simulink model "MIL_ASW"  (R2019b)
settings: Solver=FixedStepDiscrete  StartTime=0.0  StopTime=2  FixedStep=0.001  RelTol=1e-3  EnableMultiTasking=on
model workspace (MAT data in the model file):
  AccPedlCanVal : Simulink.Signal (value not decoded)
  AccPedlVal : Simulink.Signal (value not decoded)
  BrkPedlCanVal : Simulink.Signal (value not decoded)
  BrkPedlVal : Simulink.Signal (value not decoded)
  Cal1 : Simulink.Parameter (value not decoded)
  Cal10 : Simulink.Parameter (value not decoded)
  Cal11 : Simulink.Parameter (value not decoded)
  Cal12 : Simulink.Parameter (value not decoded)
  Cal2 : Simulink.Parameter (value not decoded)
  Cal3 : Simulink.Parameter (value not decoded)
  Cal4 : Simulink.Parameter (value not decoded)
  Cal5 : Simulink.Parameter (value not decoded)
  Cal6 : Simulink.Parameter (value not decoded)
  Cal7 : Simulink.Parameter (value not decoded)
  Cal8 : Simulink.Parameter (value not decoded)
  Cal9 : Simulink.Parameter (value not decoded)
  Clu1Act : Simulink.Signal (value not decoded)
  Clu1PTar : Simulink.Signal (value not decoded)
  Clu1Req : Simulink.Signal (value not decoded)
  Clu1TqTar : Simulink.Signal (value not decoded)
  Clu2Act : Simulink.Signal (value not decoded)
  Clu2PTar : Simulink.Signal (value not decoded)
  Clu2Req : Simulink.Signal (value not decoded)
  Clu2TqTar : Simulink.Signal (value not decoded)
  CluKissPtPLnch : Simulink.Parameter (value not decoded)
  CluOilTRawVal : Simulink.Signal (value not decoded)
  CluOilTVal : Simulink.Signal (value not decoded)
  CluOpenTqRatMax : Simulink.Parameter (value not decoded)
  CluPMap : Simulink.Parameter (value not decoded)
  CluPMax : Simulink.Parameter (value not decoded)
  CluPMaxGear1 : Simulink.Parameter (value not decoded)
  CluPMaxGear2 : Simulink.Parameter (value not decoded)
  CluPMaxGear3 : Simulink.Parameter (value not decoded)
  CluPMaxGear4 : Simulink.Parameter (value not decoded)
  CluPMaxGear5 : Simulink.Parameter (value not decoded)
  CluPMaxGear6 : Simulink.Parameter (value not decoded)
  CluPMaxGearR : Simulink.Parameter (value not decoded)
  CluPMin : Simulink.Parameter (value not decoded)
  CluPosnMax : Simulink.Parameter (value not decoded)
  CluSoln1IRawVal : Simulink.Signal (value not decoded)
  CluSoln1IReq : Simulink.Signal (value not decoded)
  CluSoln1IReqFlg : Simulink.Signal (value not decoded)
  CluSoln1IVal : Simulink.Signal (value not decoded)
  CluSoln1LineI : Simulink.Parameter (value not decoded)
  CluSoln1LineP : Simulink.Parameter (value not decoded)
  CluSoln1Pwm : Simulink.Signal (value not decoded)
  CluSoln2IRawVal : Simulink.Signal (value not decoded)
  CluSoln2IReq : Simulink.Signal (value not decoded)
  CluSoln2IReqFlg : Simulink.Signal (value not decoded)
  CluSoln2IVal : Simulink.Signal (value not decoded)
  CluSoln2LineI : Simulink.Parameter (value not decoded)
  CluSoln2LineP : Simulink.Parameter (value not decoded)
  CluSoln2Pwm : Simulink.Signal (value not decoded)
  CluTqMap : Simulink.Parameter (value not decoded)
  CrnkSpdRawVal : Simulink.Signal (value not decoded)
  CrnkSpdVal : Simulink.Signal (value not decoded)
  Drive_Intensity_Fuzzy : object (value not decoded)
  DrvIntenFzzy : Simulink.LookupTable (value not decoded)
  EngNIdle : Simulink.Parameter (value not decoded)
  EngNIdleMin : Simulink.Parameter (value not decoded)
  EngSpdCanVal : Simulink.Signal (value not decoded)
  EngThrCanVal : Simulink.Signal (value not decoded)
  EngTqAdd : Simulink.Parameter (value not decoded)
  EngTqCanVal : Simulink.Signal (value not decoded)
  EngTqIntvFlg : Simulink.Signal (value not decoded)
  EngTqIntvRat : Simulink.Signal (value not decoded)
  EngTqMapExtChartc : Simulink.Parameter (value not decoded)
  EngTqMapSpdIndx : Simulink.Parameter (value not decoded)
  EngTqMapThrtIndx : Simulink.Parameter (value not decoded)
  EngTqMapTqMax : Simulink.Parameter (value not decoded)
  EngTqMaxNorm : Simulink.Parameter (value not decoded)
  EngTqRef : Simulink.Parameter (value not decoded)
  EvenCluPRawVal : Simulink.Signal (value not decoded)
  EvenCluPVal : Simulink.Signal (value not decoded)
  EvenInpSpdRawVal : Simulink.Signal (value not decoded)
  EvenInpSpdVal : Simulink.Signal (value not decoded)
  FcnCallTime : Simulink.Parameter (value not decoded)
  FinalRat : Simulink.Parameter (value not decoded)
  Fork1A : Simulink.Parameter (value not decoded)
  Fork1Act : Simulink.Signal (value not decoded)
  Fork1B : Simulink.Parameter (value not decoded)
  Fork1DeltaSpdTar : Simulink.Parameter (value not decoded)
  Fork1MaxSpd1A : Simulink.Parameter (value not decoded)
  Fork1MaxSpd1B : Simulink.Parameter (value not decoded)
  Fork1MaxSpd2A : Simulink.Parameter (value not decoded)
  Fork1MaxSpd2B : Simulink.Parameter (value not decoded)
  Fork1PosnA : Simulink.Parameter (value not decoded)
  Fork1PosnB : Simulink.Parameter (value not decoded)
  Fork1PosnMaxSpd1A : Simulink.Parameter (value not decoded)
  Fork1PosnMaxSpd1B : Simulink.Parameter (value not decoded)
  Fork1PosnMaxSpd2A : Simulink.Parameter (value not decoded)
  Fork1PosnMaxSpd2B : Simulink.Parameter (value not decoded)
  Fork1PosnNeut : Simulink.Parameter (value not decoded)
  Fork1PosnNeutA : Simulink.Parameter (value not decoded)
  Fork1PosnNeutB : Simulink.Parameter (value not decoded)
  Fork1PosnRawVal : Simulink.Signal (value not decoded)
  Fork1PosnSyncA : Simulink.Parameter (value not decoded)
  Fork1PosnSyncB : Simulink.Parameter (value not decoded)
  Fork1PosnVal : Simulink.Signal (value not decoded)
  Fork1SyncTar : Simulink.Parameter (value not decoded)
  Fork2A : Simulink.Parameter (value not decoded)
  Fork2Act : Simulink.Signal (value not decoded)
  Fork2B : Simulink.Parameter (value not decoded)
  Fork2DeltaSpdTar : Simulink.Parameter (value not decoded)
  Fork2MaxSpd1A : Simulink.Parameter (value not decoded)
  Fork2MaxSpd1B : Simulink.Parameter (value not decoded)
  Fork2MaxSpd2A : Simulink.Parameter (value not decoded)
  Fork2MaxSpd2B : Simulink.Parameter (value not decoded)
  Fork2PosnA : Simulink.Parameter (value not decoded)
  Fork2PosnB : Simulink.Parameter (value not decoded)
  Fork2PosnMaxSpd1A : Simulink.Parameter (value not decoded)
  Fork2PosnMaxSpd1B : Simulink.Parameter (value not decoded)
  Fork2PosnMaxSpd2A : Simulink.Parameter (value not decoded)
  Fork2PosnMaxSpd2B : Simulink.Parameter (value not decoded)
  Fork2PosnNeut : Simulink.Parameter (value not decoded)
  Fork2PosnNeutA : Simulink.Parameter (value not decoded)
  Fork2PosnNeutB : Simulink.Parameter (value not decoded)
  Fork2PosnRawVal : Simulink.Signal (value not decoded)
  Fork2PosnSyncA : Simulink.Parameter (value not decoded)
  Fork2PosnSyncB : Simulink.Parameter (value not decoded)
  Fork2PosnVal : Simulink.Signal (value not decoded)
  Fork2SyncTar : Simulink.Parameter (value not decoded)
  Fork3A : Simulink.Parameter (value not decoded)
  Fork3Act : Simulink.Signal (value not decoded)
  Fork3B : Simulink.Parameter (value not decoded)
  Fork3DeltaSpdTar : Simulink.Parameter (value not decoded)
  Fork3MaxSpd1A : Simulink.Parameter (value not decoded)
  Fork3MaxSpd1B : Simulink.Parameter (value not decoded)
  Fork3MaxSpd2A : Simulink.Parameter (value not decoded)
  Fork3MaxSpd2B : Simulink.Parameter (value not decoded)
  Fork3PosnA : Simulink.Parameter (value not decoded)
  Fork3PosnB : Simulink.Parameter (value not decoded)
  Fork3PosnMaxSpd1A : Simulink.Parameter (value not decoded)
  Fork3PosnMaxSpd1B : Simulink.Parameter (value not decoded)
  Fork3PosnMaxSpd2A : Simulink.Parameter (value not decoded)
  Fork3PosnMaxSpd2B : Simulink.Parameter (value not decoded)
  Fork3PosnNeut : Simulink.Parameter (value not decoded)
  Fork3PosnNeutA : Simulink.Parameter (value not decoded)
  Fork3PosnNeutB : Simulink.Parameter (value not decoded)
  Fork3PosnRawVal : Simulink.Signal (value not decoded)
  Fork3PosnSyncA : Simulink.Parameter (value not decoded)
  Fork3PosnSyncB : Simulink.Parameter (value not decoded)
  Fork3PosnVal : Simulink.Signal (value not decoded)
  Fork3SyncTar : Simulink.Parameter (value not decoded)
  Fork4A : Simulink.Parameter (value not decoded)
  Fork4Act : Simulink.Signal (value not decoded)
  Fork4B : Simulink.Parameter (value not decoded)
  Fork4DeltaSpdTar : Simulink.Parameter (value not decoded)
  Fork4MaxSpd1A : Simulink.Parameter (value not decoded)
  Fork4MaxSpd1B : Simulink.Parameter (value not decoded)
  Fork4MaxSpd2A : Simulink.Parameter (value not decoded)
  Fork4MaxSpd2B : Simulink.Parameter (value not decoded)
  Fork4PosnA : Simulink.Parameter (value not decoded)
  Fork4PosnB : Simulink.Parameter (value not decoded)
  Fork4PosnMaxSpd1A : Simulink.Parameter (value not decoded)
  Fork4PosnMaxSpd1B : Simulink.Parameter (value not decoded)
  Fork4PosnMaxSpd2A : Simulink.Parameter (value not decoded)
  Fork4PosnMaxSpd2B : Simulink.Parameter (value not decoded)
  Fork4PosnNeut : Simulink.Parameter (value not decoded)
  Fork4PosnNeutA : Simulink.Parameter (value not decoded)
  Fork4PosnNeutB : Simulink.Parameter (value not decoded)
  Fork4PosnRawVal : Simulink.Signal (value not decoded)
  Fork4PosnSyncA : Simulink.Parameter (value not decoded)
  Fork4PosnSyncB : Simulink.Parameter (value not decoded)
  Fork4PosnVal : Simulink.Signal (value not decoded)
  Fork4SyncTar : Simulink.Parameter (value not decoded)
  FrntWhlRd : Simulink.Parameter (value not decoded)
  GearIdx : Simulink.Parameter (value not decoded)
  GearMax : Simulink.Parameter (value not decoded)
  GearRat : Simulink.Parameter (value not decoded)
  Launch_Engage_Fuzzy : object (value not decoded)
  LnchEngmtFzzy : Simulink.LookupTable (value not decoded)
  LubeSolnIRawVal : Simulink.Signal (value not decoded)
  LubeSolnIReq : Simulink.Signal (value not decoded)
  LubeSolnIVal : Simulink.Signal (value not decoded)
  LubeSolnLineI : Simulink.Parameter (value not decoded)
  LubeSolnLineP : Simulink.Parameter (value not decoded)
  LubeSolnPwm : Simulink.Signal (value not decoded)
  MaiLineSolnIRawVal : Simulink.Signal (value not decoded)
  MaiLineSolnIReq : Simulink.Signal (value not decoded)
  MaiLineSolnIVal : Simulink.Signal (value not decoded)
  MaiLineSolnLineI : Simulink.Parameter (value not decoded)
  MaiLineSolnLineP : Simulink.Parameter (value not decoded)
  MaiLineSolnPwm : Simulink.Signal (value not decoded)
  OddCluPRawVal : Simulink.Signal (value not decoded)
  OddCluPVal : Simulink.Signal (value not decoded)
  OddInpSpdRawVal : Simulink.Signal (value not decoded)
  OddInpSpdVal : Simulink.Signal (value not decoded)
  OutpSpdRawVal : Simulink.Signal (value not decoded)
  OutpSpdVal : Simulink.Signal (value not decoded)
  PsnsrLineP : Simulink.Parameter (value not decoded)
  PsnsrLineV : Simulink.Parameter (value not decoded)
  SftLvrCanVal : Simulink.Signal (value not decoded)
  SftLvrCfm : Simulink.Signal (value not decoded)
  SftLvrVal : Simulink.Signal (value not decoded)
  Shaft1GearAct : Simulink.Signal (value not decoded)
  Shaft1GearReq : Simulink.Signal (value not decoded)
  Shaft2GearAct : Simulink.Signal (value not decoded)
  Shaft2GearReq : Simulink.Signal (value not decoded)
  ShiftMux1SwtReq : Simulink.Signal (value not decoded)
  ShiftMux2SwtReq : Simulink.Signal (value not decoded)
  ShiftSdlEcoDwnSeln : Simulink.Parameter (value not decoded)
  ShiftSdlEcoDwnShift : Simulink.Parameter (value not decoded)
  ShiftSdlEcoUpSeln : Simulink.Parameter (value not decoded)
  ShiftSdlEcoUpShift : Simulink.Parameter (value not decoded)
  ShiftSdlPwrDwnSeln : Simulink.Parameter (value not decoded)
  ShiftSdlPwrDwnShift : Simulink.Parameter (value not decoded)
  ShiftSdlPwrUpSeln : Simulink.Parameter (value not decoded)
  ShiftSdlPwrUpShift : Simulink.Parameter (value not decoded)
  ShiftSdlSACDwnSeln : Simulink.Parameter (value not decoded)
  ShiftSdlSACDwnShift : Simulink.Parameter (value not decoded)
  ShiftSdlSACUpSeln : Simulink.Parameter (value not decoded)
  ShiftSdlSACUpShift : Simulink.Parameter (value not decoded)
  ShiftSdlThrPedlIdx : Simulink.Parameter (value not decoded)
  ShiftSoln1IRawVal : Simulink.Signal (value not decoded)
  ShiftSoln1IReq : Simulink.Signal (value not decoded)
  ShiftSoln1IVal : Simulink.Signal (value not decoded)
  ShiftSoln1LineI : Simulink.Parameter (value not decoded)
  ShiftSoln1LineP : Simulink.Parameter (value not decoded)
  ShiftSoln1Pwm : Simulink.Signal (value not decoded)
  ShiftSoln2IRawVal : Simulink.Signal (value not decoded)
  ShiftSoln2IReq : Simulink.Signal (value not decoded)
  ShiftSoln2IVal : Simulink.Signal (value not decoded)
  ShiftSoln2LineI : Simulink.Parameter (value not decoded)
  ShiftSoln2LineP : Simulink.Parameter (value not decoded)
  ShiftSoln2Pwm : Simulink.Signal (value not decoded)
  SolnOutpTRawVal : Simulink.Signal (value not decoded)
  SolnOutpTVal : Simulink.Signal (value not decoded)
  TSnsr1LineR : Simulink.Parameter (value not decoded)
  TSnsr2LineR : Simulink.Parameter (value not decoded)
  TrsmNrGearAct : Simulink.Signal (value not decoded)
  TrsmNrGearReq : Simulink.Signal (value not decoded)
  TrsmNrPreGearAct : Simulink.Signal (value not decoded)
  TrsmNrPreGearReq : Simulink.Signal (value not decoded)
  Tsnsr1LineT : Simulink.Parameter (value not decoded)
  Tsnsr2LineT : Simulink.Parameter (value not decoded)
  VehSpdCanVal : Simulink.Signal (value not decoded)
  VehSpdTrsmEstimd : Simulink.Signal (value not decoded)
  VehSpdVal : Simulink.Signal (value not decoded)
  VlvBodyTRawVal : Simulink.Signal (value not decoded)
  VlvBodyTVal : Simulink.Signal (value not decoded)
symbols that are objects in the model workspace (value not decoded): CluPMap, CluSoln1LineI, CluSoln1LineP, CluSoln2LineI, CluSoln2LineP, CluTqMap, EngNIdle, EngNIdleMin, EngTqMapThrtIndx, EngTqMapTqMax, EngTqMaxNorm, FcnCallTime, FinalRat, Fork1A, Fork1B, Fork1DeltaSpdTar, Fork1PosnA, Fork1PosnB, Fork1PosnMaxSpd1A, Fork1PosnMaxSpd1B, Fork1PosnMaxSpd2A, Fork1PosnMaxSpd2B, Fork1PosnNeut, Fork1PosnNeutA, Fork1PosnNeutB, Fork1PosnSyncA, Fork1PosnSyncB, Fork1SyncTar, Fork2A, Fork2B, Fork2DeltaSpdTar, Fork2PosnA, Fork2PosnB, Fork2PosnMaxSpd1A, Fork2PosnMaxSpd1B, Fork2PosnMaxSpd2A, Fork2PosnMaxSpd2B, Fork2PosnNeut, Fork2PosnNeutA, Fork2PosnNeutB, Fork2PosnSyncA, Fork2PosnSyncB, Fork2SyncTar, Fork3A, Fork3B, Fork3DeltaSpdTar, Fork3PosnA, Fork3PosnB, Fork3PosnMaxSpd1A, Fork3PosnMaxSpd1B, Fork3PosnMaxSpd2A, Fork3PosnMaxSpd2B, Fork3PosnNeut, Fork3PosnNeutA, Fork3PosnNeutB, Fork3PosnSyncA, Fork3PosnSyncB, Fork3SyncTar, Fork4A, Fork4B
undefined symbols (not defined in the file or in its folder): in1, out1
libraries: simulink x44, fuzblock x3
(part 6 of 10)

== system MIL_ASW/Application_Software_SHAW/ASW_DrivingStrategy/Auto_Mode_Decision/SptMod ==
  AccPedlVal : Inport
  TrsmPreNrGearAct : Inport  Port=2
  TrsmNrGearAct : Inport  Port=3
  Constant : Constant  Value=30000  OutDataTypeStr=uint16
  Constant1 : Constant  Value=0  OutDataTypeStr=uint16
  Constant2 : Constant  Value=30000  OutDataTypeStr=uint16
  Constant3 : Constant  Value=0  OutDataTypeStr=uint16
  Interval Test : simulink/Logic and Bit Operations/Interval Test  IntervalClosedRight=on  uplimit=GearMax-1  IntervalClosedLeft=on  lowlimit=1  OutDataTypeStr=uint8
  Interval Test1 : simulink/Logic and Bit Operations/Interval Test  IntervalClosedRight=on  uplimit=GearMax  IntervalClosedLeft=on  lowlimit=2  OutDataTypeStr=uint8
  Interval Test2 : simulink/Logic and Bit Operations/Interval Test  IntervalClosedRight=on  uplimit=GearMax-1  IntervalClosedLeft=on  lowlimit=1  OutDataTypeStr=uint8
  Interval Test3 : simulink/Logic and Bit Operations/Interval Test  IntervalClosedRight=on  uplimit=GearMax  IntervalClosedLeft=on  lowlimit=2  OutDataTypeStr=uint8
  Saturation : Saturate  UpperLimit=GearMax-1  LowerLimit=1  OutDataTypeStr=uint8
  Saturation1 : Saturate  UpperLimit=GearMax  LowerLimit=2  OutDataTypeStr=uint8
  Saturation2 : Saturate  UpperLimit=GearMax-1  LowerLimit=1  OutDataTypeStr=uint8
  Saturation3 : Saturate  UpperLimit=GearMax  LowerLimit=2  OutDataTypeStr=uint8
  Select{1..4} (4 alike) : Switch  Criteria=u2 ~= 0
  ShiftSdlPwrDwnSeln : Lookup_n-D  BreakpointsForDimension1=ShiftSdlThrPedlIdx  BreakpointsForDimension2=GearIdx  Table=ShiftSdlPwrDwnSeln  TableDataTypeStr=uint16  ExtrapMethod=Clip  OutDataTypeStr=Inherit: Inherit from 'Table data'  RndMeth=Simplest  InputSameDT=on
  ShiftSdlPwrDwnShift : Lookup_n-D  BreakpointsForDimension1=ShiftSdlThrPedlIdx  BreakpointsForDimension2=GearIdx  Table=ShiftSdlPwrDwnShift  TableDataTypeStr=uint16  ExtrapMethod=Clip  OutDataTypeStr=Inherit: Inherit from 'Table data'  RndMeth=Simplest  InputSameDT=on
  ShiftSdlPwrUpSeln : Lookup_n-D  BreakpointsForDimension1=ShiftSdlThrPedlIdx  BreakpointsForDimension2=GearIdx  Table=ShiftSdlPwrUpSeln  TableDataTypeStr=uint16  ExtrapMethod=Clip  OutDataTypeStr=Inherit: Inherit from 'Table data'  RndMeth=Simplest  InputSameDT=on
  ShiftSdlPwrUpShift : Lookup_n-D  BreakpointsForDimension1=ShiftSdlThrPedlIdx  BreakpointsForDimension2=GearIdx  Table=ShiftSdlPwrUpShift  TableDataTypeStr=uint16  ExtrapMethod=Clip  OutDataTypeStr=Inherit: Inherit from 'Table data'  RndMeth=Simplest  InputSameDT=on
  u-1 : Subsystem
  u-2 : Subsystem
  UpSeln : Outport  VectorParamsAs1DForOutWhenUnconnected=off
  DwnSeln : Outport  Port=2  VectorParamsAs1DForOutWhenUnconnected=off
  UpShift : Outport  Port=3  VectorParamsAs1DForOutWhenUnconnected=off
  DwnShift : Outport  Port=4  VectorParamsAs1DForOutWhenUnconnected=off
  wires:
  TrsmPreNrGearAct/1 -> Saturation/1, Interval Test/1, Saturation1/1, Interval Test1/1
  u-1/1(Out) -> ShiftSdlPwrDwnShift/2
  u-2/1(Out) -> ShiftSdlPwrDwnSeln/2
  AccPedlVal/1 -> ShiftSdlPwrDwnSeln/1, ShiftSdlPwrUpShift/1, ShiftSdlPwrDwnShift/1, ShiftSdlPwrUpSeln/1
  ShiftSdlPwrUpSeln/1 -> Select1/1
  ShiftSdlPwrDwnSeln/1 -> Select2/1
  ShiftSdlPwrUpShift/1 -> Select3/1
  ShiftSdlPwrDwnShift/1 -> Select4/1
  Interval Test/1 -> Select1/2
  Interval Test1/1 -> Select2/2
  Interval Test2/1 -> Select3/2
  Interval Test3/1 -> Select4/2
  Constant/1 -> Select1/3
  Constant1/1 -> Select2/3
  Constant2/1 -> Select3/3
  Constant3/1 -> Select4/3
  Select1/1 -> UpSeln/1
  Select2/1 -> DwnSeln/1
  Select3/1 -> UpShift/1
  Select4/1 -> DwnShift/1
  Saturation/1 -> ShiftSdlPwrUpSeln/2
  Saturation2/1 -> ShiftSdlPwrUpShift/2
  Saturation1/1 -> u-2/1(In)
  Saturation3/1 -> u-1/1(In)
  TrsmNrGearAct/1 -> Interval Test2/1, Saturation3/1, Interval Test3/1, Saturation2/1

== system MIL_ASW/Application_Software_SHAW/ASW_DrivingStrategy/Auto_Mode_Decision/TrsmNrGearTarCalcnAutMod/Upshift_Frozen ==
  acc_pedl : Inport  OutDataTypeStr=uint8
  brk_pedl : Inport  Port=2  OutDataTypeStr=uint8
  veh_spd : Inport  Port=3  OutDataTypeStr=uint16
  f : TriggerPort  TriggerType=function-call  VariantControl=(inherit)
      settings: CopyFcn=Stateflow.SLINSF.SimulinkMan.removeBlockPreDeleteFcn  PreDeleteFcn=Stateflow.SLINSF.SimulinkMan.unsafePredeleteFcn
  Compare To Zero : simulink/Logic and Bit Operations/Compare To Zero  relop=<=  OutDataTypeStr=boolean
  Compare To Zero1 : simulink/Logic and Bit Operations/Compare To Zero  relop=>  OutDataTypeStr=boolean
  Constant : Constant  OutDataTypeStr=uint8
  Constant1 : Constant  Value=0  OutDataTypeStr=uint8
  Delay : Delay  DelayLength=1  InitialCondition=0
  Delay1 : Delay  InitialCondition=0
  Delay2 : Delay  DelayLength=10  InitialCondition=0
  Logical Operator : Logic  Operator=OR  Inputs=3  AllPortsSameDT=off  OutDataTypeStr=boolean
  Logical Operator1 : Logic  Operator=OR  Inputs=3  AllPortsSameDT=off  OutDataTypeStr=boolean
  Logical Operator2 : Logic  Operator=NOR  Inputs=3  AllPortsSameDT=off  OutDataTypeStr=boolean
  Relational Operator : RelationalOperator  Operator=<  OutDataTypeStr=boolean  RndMeth=Simplest
  Relational Operator1 : RelationalOperator  Operator=<  OutDataTypeStr=boolean  RndMeth=Simplest
  Relational Operator2 : RelationalOperator  Operator=<  OutDataTypeStr=boolean  RndMeth=Simplest
  Switch : Switch  Criteria=u2 > Threshold
  Switch1 : Switch  Criteria=u2 > Threshold
  Terminator : Terminator
  Unit Delay1 : UnitDelay  SampleTime=-1  HasFrameUpgradeWarning=on
  flag : Outport  OutDataTypeStr=uint8  VectorParamsAs1DForOutWhenUnconnected=off
  wires:
  Delay/1 -> Relational Operator/2
  Switch/1 -> Unit Delay1/1, flag/1
  Constant/1 -> Switch/1
  Switch1/1 -> Switch/3
  veh_spd/1 -> Terminator/1
  Logical Operator2/1 -> Switch1/2
  Constant1/1 -> Switch1/1
  Unit Delay1/1 -> Switch1/3
  Delay1/1 -> Relational Operator1/2
  Delay2/1 -> Relational Operator2/2
  acc_pedl/1 -> Relational Operator2/1, Compare To Zero/1, Delay2/1, Delay1/1, Relational Operator1/1, Delay/1, Relational Operator/1
  Relational Operator/1 -> Logical Operator/1
  Relational Operator1/1 -> Logical Operator/2
  Relational Operator2/1 -> Logical Operator/3
  Compare To Zero/1 -> Logical Operator2/2, Logical Operator1/2
  brk_pedl/1 -> Compare To Zero1/1
  Logical Operator/1 -> Logical Operator2/1, Logical Operator1/1
  Compare To Zero1/1 -> Logical Operator2/3, Logical Operator1/3
  Logical Operator1/1 -> Switch/2

== system MIL_ASW/Application_Software_SHAW/ASW_GearPositioner/Fork1/Ini_ForkAct/position_A ==
  In1 : Inport
  Action Port : ActionPort  ActionPortLabel=elseif(u1>u2)
  Out1 : Outport  VectorParamsAs1DForOutWhenUnconnected=off
  wires:
  In1/1 -> Out1/1

== system MIL_ASW/Application_Software_SHAW/ASW_GearPositioner/Fork1/Ini_ForkAct/position_B ==
  In1 : Inport
  Action Port : ActionPort  ActionPortLabel=elseif( u1<u5)
  Out1 : Outport  VectorParamsAs1DForOutWhenUnconnected=off
  wires:
  In1/1 -> Out1/1

== system MIL_ASW/Application_Software_SHAW/ASW_GearPositioner/Fork1/Ini_ForkAct/position_between_Neutral_A ==
  In1 : Inport
  Action Port : ActionPort  ActionPortLabel=elseif( u1<=u2&u1>u3)
  Out1 : Outport  VectorParamsAs1DForOutWhenUnconnected=off
  wires:
  In1/1 -> Out1/1

== system MIL_ASW/Application_Software_SHAW/ASW_GearPositioner/Fork1/Ini_ForkAct/position_between_Neutral_B ==
  In1 : Inport
  Action Port : ActionPort  ActionPortLabel=elseif( u1<u4&u1>=u5)
  Out1 : Outport  VectorParamsAs1DForOutWhenUnconnected=off
  wires:
  In1/1 -> Out1/1

== system MIL_ASW/Application_Software_SHAW/ASW_GearPositioner/Fork1/Ini_ForkAct/position_neutral ==
  In1 : Inport
  Action Port : ActionPort  ActionPortLabel=if(u1<=u3&u1>=u4)
  Out1 : Outport  VectorParamsAs1DForOutWhenUnconnected=off
  wires:
  In1/1 -> Out1/1

== system MIL_ASW/Application_Software_SHAW/ASW_GearPositioner/Fork2/Ini_ForkAct/position_A ==
  In1 : Inport
  Action Port : ActionPort  ActionPortLabel=elseif(u1>u2)
  Out1 : Outport  VectorParamsAs1DForOutWhenUnconnected=off
  wires:
  In1/1 -> Out1/1

== system MIL_ASW/Application_Software_SHAW/ASW_GearPositioner/Fork2/Ini_ForkAct/position_B ==
  In1 : Inport
  Action Port : ActionPort  ActionPortLabel=elseif( u1<u5)
  Out1 : Outport  VectorParamsAs1DForOutWhenUnconnected=off
  wires:
  In1/1 -> Out1/1

== system MIL_ASW/Application_Software_SHAW/ASW_GearPositioner/Fork2/Ini_ForkAct/position_between_Neutral_A ==
  In1 : Inport
  Action Port : ActionPort  ActionPortLabel=elseif( u1<=u2&u1>u3)
  Out1 : Outport  VectorParamsAs1DForOutWhenUnconnected=off
  wires:
  In1/1 -> Out1/1

== system MIL_ASW/Application_Software_SHAW/ASW_GearPositioner/Fork2/Ini_ForkAct/position_between_Neutral_B ==
  In1 : Inport
  Action Port : ActionPort  ActionPortLabel=elseif( u1<u4&u1>=u5)
  Out1 : Outport  VectorParamsAs1DForOutWhenUnconnected=off
  wires:
  In1/1 -> Out1/1

== system MIL_ASW/Application_Software_SHAW/ASW_GearPositioner/Fork2/Ini_ForkAct/position_neutral ==
  In1 : Inport
  Action Port : ActionPort  ActionPortLabel=if(u1<=u3&u1>=u4)
  Out1 : Outport  VectorParamsAs1DForOutWhenUnconnected=off
  wires:
  In1/1 -> Out1/1

== system MIL_ASW/Application_Software_SHAW/ASW_GearPositioner/Fork3/Ini_ForkAct/position_A ==
  In1 : Inport
  Action Port : ActionPort  ActionPortLabel=elseif(u1>u2)
  Out1 : Outport  VectorParamsAs1DForOutWhenUnconnected=off
  wires:
  In1/1 -> Out1/1

== system MIL_ASW/Application_Software_SHAW/ASW_GearPositioner/Fork3/Ini_ForkAct/position_B ==
  In1 : Inport
  Action Port : ActionPort  ActionPortLabel=elseif( u1<u5)
  Out1 : Outport  VectorParamsAs1DForOutWhenUnconnected=off
  wires:
  In1/1 -> Out1/1

== system MIL_ASW/Application_Software_SHAW/ASW_GearPositioner/Fork3/Ini_ForkAct/position_between_Neutral_A ==
  In1 : Inport
  Action Port : ActionPort  ActionPortLabel=elseif( u1<=u2&u1>u3)
  Out1 : Outport  VectorParamsAs1DForOutWhenUnconnected=off
  wires:
  In1/1 -> Out1/1

== system MIL_ASW/Application_Software_SHAW/ASW_GearPositioner/Fork3/Ini_ForkAct/position_between_Neutral_B ==
  In1 : Inport
  Action Port : ActionPort  ActionPortLabel=elseif( u1<u4&u1>=u5)
  Out1 : Outport  VectorParamsAs1DForOutWhenUnconnected=off
  wires:
  In1/1 -> Out1/1

== system MIL_ASW/Application_Software_SHAW/ASW_GearPositioner/Fork3/Ini_ForkAct/position_neutral ==
  In1 : Inport
  Action Port : ActionPort  ActionPortLabel=if(u1<=u3&u1>=u4)
  Out1 : Outport  VectorParamsAs1DForOutWhenUnconnected=off
  wires:
  In1/1 -> Out1/1

== system MIL_ASW/Application_Software_SHAW/ASW_GearPositioner/Fork4/Ini_ForkAct/position_A ==
  In1 : Inport
  Action Port : ActionPort  ActionPortLabel=elseif(u1>u2)
  Out1 : Outport  VectorParamsAs1DForOutWhenUnconnected=off
  wires:
  In1/1 -> Out1/1

== system MIL_ASW/Application_Software_SHAW/ASW_GearPositioner/Fork4/Ini_ForkAct/position_B ==
  In1 : Inport
  Action Port : ActionPort  ActionPortLabel=elseif( u1<u5)
  Out1 : Outport  VectorParamsAs1DForOutWhenUnconnected=off
  wires:
  In1/1 -> Out1/1

== system MIL_ASW/Application_Software_SHAW/ASW_GearPositioner/Fork4/Ini_ForkAct/position_between_Neutral_A ==
  In1 : Inport
  Action Port : ActionPort  ActionPortLabel=elseif( u1<=u2&u1>u3)
  Out1 : Outport  VectorParamsAs1DForOutWhenUnconnected=off
  wires:
  In1/1 -> Out1/1

== system MIL_ASW/Application_Software_SHAW/ASW_GearPositioner/Fork4/Ini_ForkAct/position_between_Neutral_B ==
  In1 : Inport
  Action Port : ActionPort  ActionPortLabel=elseif( u1<u4&u1>=u5)
  Out1 : Outport  VectorParamsAs1DForOutWhenUnconnected=off
  wires:
  In1/1 -> Out1/1

== system MIL_ASW/Application_Software_SHAW/ASW_GearPositioner/Fork4/Ini_ForkAct/position_neutral ==
  In1 : Inport
  Action Port : ActionPort  ActionPortLabel=if(u1<=u3&u1>=u4)
  Out1 : Outport  VectorParamsAs1DForOutWhenUnconnected=off
  wires:
  In1/1 -> Out1/1

== system MIL_ASW/Application_Software_SHAW/ASW_GearPositioner/SpdSwicht/Substrate1 ==
  In1 : Inport
  In2 : Inport  Port=2
  Add : Sum  Inputs=+-
  Logical Operator : Logic  Operator=NOT  AllPortsSameDT=off  OutDataTypeStr=boolean
  Relational Operator : RelationalOperator  OutDataTypeStr=boolean  RndMeth=Nearest
  Switch : Switch  Criteria=u2 ~= 0  OutDataTypeStr=uint16
  Switch1 : Switch  Criteria=u2 ~= 0  OutDataTypeStr=uint16
  Out1 : Outport  VectorParamsAs1DForOutWhenUnconnected=off
  wires:
  Add/1 -> Out1/1
  In1/1 -> Switch1/1, Switch/1, Relational Operator/1
  In2/1 -> Relational Operator/2, Switch/3, Switch1/3
  Relational Operator/1 -> Logical Operator/1, Switch/2
  Switch/1 -> Add/1
  Logical Operator/1 -> Switch1/2
  Switch1/1 -> Add/2

== system MIL_ASW/Application_Software_SHAW/ASW_GearPositioner/SpdSwicht/Substrate2 ==
  In1 : Inport
  In2 : Inport  Port=2
  Add : Sum  Inputs=+-
  Logical Operator : Logic  Operator=NOT  AllPortsSameDT=off  OutDataTypeStr=boolean
  Relational Operator : RelationalOperator  OutDataTypeStr=boolean  RndMeth=Nearest
  Switch : Switch  Criteria=u2 ~= 0  OutDataTypeStr=uint16
  Switch1 : Switch  Criteria=u2 ~= 0  OutDataTypeStr=uint16
  Out1 : Outport  VectorParamsAs1DForOutWhenUnconnected=off
  wires:
  Switch1/1 -> Add/2
  Logical Operator/1 -> Switch1/2
  Switch/1 -> Add/1
  Relational Operator/1 -> Switch/2, Logical Operator/1
  In2/1 -> Switch1/3, Switch/3, Relational Operator/2
  In1/1 -> Relational Operator/1, Switch/1, Switch1/1
  Add/1 -> Out1/1

== system MIL_ASW/Application_Software_SHAW/ASW_GearPositioner/SpdSwicht/Substrate3 ==
  In1 : Inport
  In2 : Inport  Port=2
  Add : Sum  Inputs=+-
  Logical Operator : Logic  Operator=NOT  AllPortsSameDT=off  OutDataTypeStr=boolean
  Relational Operator : RelationalOperator  OutDataTypeStr=boolean  RndMeth=Nearest
  Switch : Switch  Criteria=u2 ~= 0  OutDataTypeStr=uint16
  Switch1 : Switch  Criteria=u2 ~= 0  OutDataTypeStr=uint16
  Out1 : Outport  VectorParamsAs1DForOutWhenUnconnected=off
  wires:
  Add/1 -> Out1/1
  In1/1 -> Switch1/1, Switch/1, Relational Operator/1
  In2/1 -> Relational Operator/2, Switch/3, Switch1/3
  Relational Operator/1 -> Logical Operator/1, Switch/2
  Switch/1 -> Add/1
  Logical Operator/1 -> Switch1/2
  Switch1/1 -> Add/2

== system MIL_ASW/Application_Software_SHAW/ASW_GearPositioner/SpdSwicht/Substrate5 ==
  In1 : Inport
  In2 : Inport  Port=2
  Add : Sum  Inputs=+-
  Logical Operator : Logic  Operator=NOT  AllPortsSameDT=off  OutDataTypeStr=boolean
  Relational Operator : RelationalOperator  OutDataTypeStr=boolean  RndMeth=Nearest
  Switch : Switch  Criteria=u2 ~= 0  OutDataTypeStr=uint16
  Switch1 : Switch  Criteria=u2 ~= 0  OutDataTypeStr=uint16
  Out1 : Outport  VectorParamsAs1DForOutWhenUnconnected=off
  wires:
  Add/1 -> Out1/1
  In1/1 -> Switch1/1, Switch/1, Relational Operator/1
  In2/1 -> Relational Operator/2, Switch/3, Switch1/3
  Relational Operator/1 -> Logical Operator/1, Switch/2
  Switch/1 -> Add/1
  Logical Operator/1 -> Switch1/2
  Switch1/1 -> Add/2

== system MIL_ASW/Application_Software_SHAW/ASW_GearPositioner/SpdSwicht/Substrate6 ==
  In1 : Inport
  In2 : Inport  Port=2
  Add : Sum  Inputs=+-
  Logical Operator : Logic  Operator=NOT  AllPortsSameDT=off  OutDataTypeStr=boolean
  Relational Operator : RelationalOperator  OutDataTypeStr=boolean  RndMeth=Nearest
  Switch : Switch  Criteria=u2 ~= 0  OutDataTypeStr=uint16
  Switch1 : Switch  Criteria=u2 ~= 0  OutDataTypeStr=uint16
  Out1 : Outport  VectorParamsAs1DForOutWhenUnconnected=off
  wires:
  Switch1/1 -> Add/2
  Logical Operator/1 -> Switch1/2
  Switch/1 -> Add/1
  Relational Operator/1 -> Switch/2, Logical Operator/1
  In2/1 -> Switch1/3, Switch/3, Relational Operator/2
  In1/1 -> Relational Operator/1, Switch/1, Switch1/1
  Add/1 -> Out1/1

== system MIL_ASW/Application_Software_SHAW/ASW_GearPositioner/SpdSwicht/Substrate7 ==
  In1 : Inport
  In2 : Inport  Port=2
  Add : Sum  Inputs=+-
  Logical Operator : Logic  Operator=NOT  AllPortsSameDT=off  OutDataTypeStr=boolean
  Relational Operator : RelationalOperator  OutDataTypeStr=boolean  RndMeth=Nearest
  Switch : Switch  Criteria=u2 ~= 0  OutDataTypeStr=uint16
  Switch1 : Switch  Criteria=u2 ~= 0  OutDataTypeStr=uint16
  Out1 : Outport  VectorParamsAs1DForOutWhenUnconnected=off
  wires:
  Add/1 -> Out1/1
  In1/1 -> Switch1/1, Switch/1, Relational Operator/1
  In2/1 -> Relational Operator/2, Switch/3, Switch1/3
  Relational Operator/1 -> Logical Operator/1, Switch/2
  Switch/1 -> Add/1
  Logical Operator/1 -> Switch1/2
  Switch1/1 -> Add/2

== system MIL_ASW/Application_Software_SHAW/ASW_GearPositioner/SpdSwicht/Substrate8 ==
  In1 : Inport
  In2 : Inport  Port=2
  Add : Sum  Inputs=+-
  Logical Operator : Logic  Operator=NOT  AllPortsSameDT=off  OutDataTypeStr=boolean
  Relational Operator : RelationalOperator  OutDataTypeStr=boolean  RndMeth=Nearest
  Switch : Switch  Criteria=u2 ~= 0  OutDataTypeStr=uint16
  Switch1 : Switch  Criteria=u2 ~= 0  OutDataTypeStr=uint16
  Out1 : Outport  VectorParamsAs1DForOutWhenUnconnected=off
  wires:
  Switch1/1 -> Add/2
  Logical Operator/1 -> Switch1/2
  Switch/1 -> Add/1
  Relational Operator/1 -> Switch/2, Logical Operator/1
  In2/1 -> Switch1/3, Switch/3, Relational Operator/2
  In1/1 -> Relational Operator/1, Switch/1, Switch1/1
  Add/1 -> Out1/1

== system MIL_ASW/Application_Software_SHAW/ASW_DrivingStrategy/Auto_Mode_Decision/EcoMod/u-1 ==
  In : Inport
  Constant4 : Constant  OutDataTypeStr=uint8
  Sum : Sum  Inputs=+-  OutDataTypeStr=uint8  SaturateOnIntegerOverflow=on
  Out : Outport  VectorParamsAs1DForOutWhenUnconnected=off
  wires:
  Sum/1 -> Out/1
  In/1 -> Sum/1
  Constant4/1 -> Sum/2

== system MIL_ASW/Application_Software_SHAW/ASW_DrivingStrategy/Auto_Mode_Decision/EcoMod/u-2 ==
  In : Inport
  Constant4 : Constant  OutDataTypeStr=uint8
  Sum : Sum  Inputs=+-  OutDataTypeStr=uint8  SaturateOnIntegerOverflow=on
  Out : Outport  VectorParamsAs1DForOutWhenUnconnected=off
  wires:
  Constant4/1 -> Sum/2
  In/1 -> Sum/1
  Sum/1 -> Out/1

== system MIL_ASW/Application_Software_SHAW/ASW_DrivingStrategy/Auto_Mode_Decision/SAC_Original/u-1 ==
  In : Inport
  Constant4 : Constant  OutDataTypeStr=uint8
  Sum : Sum  Inputs=+-  OutDataTypeStr=uint8  SaturateOnIntegerOverflow=on
  Out : Outport  VectorParamsAs1DForOutWhenUnconnected=off
  wires:
  Sum/1 -> Out/1
  In/1 -> Sum/1
  Constant4/1 -> Sum/2

== system MIL_ASW/Application_Software_SHAW/ASW_DrivingStrategy/Auto_Mode_Decision/SAC_Original/u-2 ==
  In : Inport
  Constant4 : Constant  OutDataTypeStr=uint8
  Sum : Sum  Inputs=+-  OutDataTypeStr=uint8  SaturateOnIntegerOverflow=on
  Out : Outport  VectorParamsAs1DForOutWhenUnconnected=off
  wires:
  Constant4/1 -> Sum/2
  In/1 -> Sum/1
  Sum/1 -> Out/1

== system MIL_ASW/Application_Software_SHAW/ASW_DrivingStrategy/Auto_Mode_Decision/SptMod/u-1 ==
  In : Inport
  Constant4 : Constant  OutDataTypeStr=uint8
  Sum : Sum  Inputs=+-  OutDataTypeStr=uint8  SaturateOnIntegerOverflow=on
  Out : Outport  VectorParamsAs1DForOutWhenUnconnected=off
  wires:
  Constant4/1 -> Sum/2
  In/1 -> Sum/1
  Sum/1 -> Out/1

== system MIL_ASW/Application_Software_SHAW/ASW_DrivingStrategy/Auto_Mode_Decision/SptMod/u-2 ==
  In : Inport
  Constant4 : Constant  OutDataTypeStr=uint8
  Sum : Sum  Inputs=+-  OutDataTypeStr=uint8  SaturateOnIntegerOverflow=on
  Out : Outport  VectorParamsAs1DForOutWhenUnconnected=off
  wires:
  Sum/1 -> Out/1
  In/1 -> Sum/1
  Constant4/1 -> Sum/2

== stateflow chart MIL_ASW/Application_Software_SHAW/ASW_GearPositioner/Fork2 ==
  state PosnTar = PosnTar(PosnAct) [function]
  state ForkAct = Ini_ForkAct(PosnAct) [function]
  state Initialization
    en:
    Fork2DirReq=0;
    Fork2PosnReq=Fork2PosnVal;
    du:
    Fork2ActLoc=Ini_ForkAct(Fork2PosnVal);
    ex:
    Fork2PosnReq=Fork2PosnVal;
  state error1
  state error
  state PositionBEngage
    state Phase1
      en,du:
      Fork2SyncPha=1;
      Fork2PosnReq=Fork2PosnVal-PosnTar(Fork2PosnVal);
    state Phase2
      en,du:
      Fork2SyncPha=2;
      Fork2DeltaSpdAct=Fork2BDeltaSpdAct;
      Fork2DeltaSpdReq=Fork2DeltaSpdAct-Fork2DeltaSpdTar*FcnCallTime;
    state Phase3
      en,du:
      Fork2SyncPha=3;
      Fork2PosnReq=Fork2PosnVal-PosnTar(Fork2PosnVal);
    PositionBEngage.Phase1 -> PositionBEngage.Phase2 : [Fork2PosnReq<=Fork2PosnSyncB]
    PositionBEngage.Phase2 -> PositionBEngage.Phase3 : [Fork2DeltaSpdAct<=Fork2SyncTar]
  state PositionAEngage
    state Phase1
      en,du:
      Fork2SyncPha=1;
      Fork2PosnReq=Fork2PosnVal+PosnTar(Fork2PosnVal);
    state Phase2
      en,du:
      Fork2SyncPha=2;
      Fork2DeltaSpdAct=Fork2ADeltaSpdAct;
      Fork2DeltaSpdReq=Fork2DeltaSpdAct-Fork2DeltaSpdTar*FcnCallTime;
    state Phase3
      en,du:
      Fork2SyncPha=3;
      Fork2PosnReq=Fork2PosnVal+PosnTar(Fork2PosnVal);
    PositionAEngage.Phase1 -> PositionAEngage.Phase2 : [Fork2PosnVal>=Fork2PosnSyncA]
    PositionAEngage.Phase2 -> PositionAEngage.Phase3 : [Fork2DeltaSpdAct<=Fork2SyncTar]
  state PositionADisengage
    state Phase1
      en:
      Fork2SyncPha=4;
      Fork2PosnReq=Fork2PosnNeut;
  state PositionBDisengage
    state Phase1
      en:
      Fork2SyncPha=4;
      Fork2PosnReq=Fork2PosnNeut;
  state Finish
    en:
    Fork2DirReq=0;
    Fork2ActLoc=Fork2ReqLoc;
    Fork2Act=Fork2ReqLoc;
  state Finish1
    en:
    Fork2DirReq=0;
    Fork2ActLoc=Fork2ReqLoc;
    Fork2Act=Fork2ReqLoc;
  (default) -> Initialization
  (junction 105) -> Initialization
  (junction 145) -> Initialization
  (junction 183) -> (junction 105)
  (junction 177) -> (junction 145)
  Initialization -> (junction 19) : [Fork2Req!=Fork2ActLoc]{Fork2ReqLoc=Fork2Req;}
  error -> (junction 177)
  (junction 21) -> error1 [order 3] : [Fork2ActLoc!=0]
  (junction 19) -> (junction 21) [order 2]
  (junction 19) -> (junction 22) [order 1] : [Fork2ReqLoc==0]
  (junction 22) -> error [order 3]
  error1 -> (junction 183)
  (junction 146) -> (junction 177)
  (junction 22) -> (junction 132) [order 1] : [Fork2ActLoc==Fork2A||...
      | Fork2ActLoc==Fork2A*10]
  (junction 21) -> (junction 27) [order 2] : [Fork2ReqLoc==Fork2B]
  (junction 21) -> (junction 72) [order 1] : [Fork2ReqLoc==Fork2A]
  (junction 22) -> (junction 131) [order 2] : [Fork2ActLoc==Fork2B||...
      | Fork2ActLoc==Fork2B*10]
  (junction 106) -> (junction 183)
  (junction 27) -> PositionBEngage.Phase1 : {Fork2DirReq=3;}
  (junction 131) -> PositionBDisengage.Phase1 : {Fork2DirReq=2;}
  (junction 72) -> PositionAEngage.Phase1 : {Fork2DirReq=1;}
  (junction 132) -> PositionADisengage.Phase1 : {Fork2DirReq=4;}
  Finish -> (junction 106)
  Finish1 -> (junction 146)
  PositionAEngage.Phase3 -> Finish : [Fork2PosnVal>=Fork2PosnA]
      | {Fork2SyncPha=4;}
  PositionBDisengage.Phase1 -> Finish1 : [Fork2PosnVal>=Fork2PosnNeutB]
      | {Fork2SyncPha=0;}
  PositionBEngage.Phase3 -> Finish : [Fork2PosnVal<=Fork2PosnB]
      | {Fork2SyncPha=4;}
  PositionADisengage.Phase1 -> Finish1 : [Fork2PosnVal<=Fork2PosnNeutA]
      | {Fork2SyncPha=0;}
  data: PosnTar function_output; PosnAct function_input uint16; PosnAct function_input uint16; ForkAct function_output; Fork2DirReq output uint8; Fork2SyncPha output uint8; Fork2DeltaSpdReq output uint16; Fork2PosnReq output uint16; Fork2DeltaSpdAct output uint16; Fork2Req input uint8; Fork2Act output uint8; Fork2PosnVal input uint16; Fork2ADeltaSpdAct input uint16; Fork2A parameter uint8; Fork2B parameter uint8; Fork2PosnSyncA parameter uint16; Fork2PosnSyncB parameter uint16; Fork2SyncTar parameter uint16; Fork2ReqLoc local uint8; Fork2DeltaSpdTar parameter uint16; FcnCallTime parameter uint8; Fork2PosnA parameter uint16; Fork2PosnB parameter uint16; Fork2PosnNeut parameter uint16; Fork2PosnNeutB parameter uint16; Fork2PosnNeutA parameter uint16; Fork2BDeltaSpdAct input uint16; Fork2ActLoc local uint8

== stateflow chart MIL_ASW/Application_Software_SHAW/ASW_GearPositioner/Fork3 ==
  state PosnTar = PosnTar(ForkAct) [function]
  state ForkAct = Ini_ForkAct(PosnAct) [function]
  state Initialization
    en:
    Fork3DirReq=0;
    Fork3PosnReq=Fork3PosnVal;
    du:
    Fork3ActLoc=Ini_ForkAct(Fork3PosnVal);
    ex:
    Fork3PosnReq=Fork3PosnVal;
  state error1
  state error
  state PositionBEngage
    state Phase1
      en,du:
      Fork3SyncPha=1;
      Fork3PosnReq=Fork3PosnVal-PosnTar(Fork3PosnVal);
    state Phase2
      en,du:
      Fork3SyncPha=2;
      Fork3DeltaSpdAct=Fork3BDeltaSpdAct;
      Fork3DeltaSpdReq=Fork3DeltaSpdAct-Fork3DeltaSpdTar*FcnCallTime;
    state Phase3
      en,du:
      Fork3SyncPha=3;
      Fork3PosnReq=Fork3PosnVal-PosnTar(Fork3PosnVal);
    PositionBEngage.Phase1 -> PositionBEngage.Phase2 : [Fork3PosnReq<=Fork3PosnSyncB]
    PositionBEngage.Phase2 -> PositionBEngage.Phase3 : [Fork3DeltaSpdAct<=Fork3SyncTar]
  state PositionAEngage
    state Phase1
      en,du:
      Fork3SyncPha=1;
      Fork3PosnReq=Fork3PosnVal+PosnTar(Fork3PosnVal);
    state Phase2
      en,du:
      Fork3SyncPha=2;
      Fork3DeltaSpdAct=Fork3ADeltaSpdAct;
      Fork3DeltaSpdReq=Fork3DeltaSpdAct-Fork3DeltaSpdTar*FcnCallTime;
    state Phase3
      en,du:
      Fork3SyncPha=3;
      Fork3PosnReq=Fork3PosnVal+PosnTar(Fork3PosnVal);
    PositionAEngage.Phase1 -> PositionAEngage.Phase2 : [Fork3PosnVal>=Fork3PosnSyncA]
    PositionAEngage.Phase2 -> PositionAEngage.Phase3 : [Fork3DeltaSpdAct<=Fork3SyncTar]
  state PositionADisengage
    state Phase1
      en:
      Fork3SyncPha=4;
      Fork3PosnReq=Fork3PosnNeut;
  state PositionBDisengage
    state Phase1
      en:
      Fork3SyncPha=4;
      Fork3PosnReq=Fork3PosnNeut;
  state Finish
    en:
    Fork3DirReq=0;
    Fork3ActLoc=Fork3ReqLoc;
    Fork3Act=Fork3ReqLoc;
  state Finish1
    en:
    Fork3DirReq=0;
    Fork3ActLoc=Fork3ReqLoc;
    Fork3Act=Fork3ReqLoc;
  (default) -> Initialization
  (junction 105) -> Initialization
  (junction 145) -> Initialization
  (junction 183) -> (junction 105)
  (junction 177) -> (junction 145)
  Initialization -> (junction 19) : [Fork3Req!=Fork3ActLoc]{Fork3ReqLoc=Fork3Req;}
  error -> (junction 177)
  (junction 21) -> error1 [order 3] : [Fork3ActLoc!=0]
  (junction 19) -> (junction 21) [order 2]
  (junction 19) -> (junction 22) [order 1] : [Fork3ReqLoc==0]
  (junction 22) -> error [order 3]
  error1 -> (junction 183)
  (junction 146) -> (junction 177)
  (junction 22) -> (junction 132) [order 1] : [Fork3ActLoc==Fork3A||...
      | Fork3ActLoc==Fork3A*10]
  (junction 21) -> (junction 27) [order 2] : [Fork3ReqLoc==Fork3B]
  (junction 21) -> (junction 72) [order 1] : [Fork3ReqLoc==Fork3A]
  (junction 22) -> (junction 131) [order 2] : [Fork3ActLoc==Fork3B||...
      | Fork3ActLoc==Fork3B*10]
  (junction 106) -> (junction 183)
  (junction 27) -> PositionBEngage.Phase1 : {Fork3DirReq=3;}
  (junction 131) -> PositionBDisengage.Phase1 : {Fork3DirReq=2;}
  (junction 132) -> PositionADisengage.Phase1 : {Fork3DirReq=4;}
  (junction 72) -> PositionAEngage.Phase1 : {Fork3DirReq=1;}
  Finish -> (junction 106)
  Finish1 -> (junction 146)
  PositionBDisengage.Phase1 -> Finish1 : [Fork3PosnVal>=Fork3PosnNeutB]
      | {Fork3SyncPha=0;}
  PositionBEngage.Phase3 -> Finish : [Fork3PosnVal<=Fork3PosnB]
      | {Fork3SyncPha=4;}
  PositionADisengage.Phase1 -> Finish1 : [Fork3PosnVal<=Fork3PosnNeutA]
      | {Fork3SyncPha=0;}
  PositionAEngage.Phase3 -> Finish : [Fork3PosnVal>=Fork3PosnA]
      | {Fork3SyncPha=4;}
  data: PosnTar function_output; ForkAct function_input uint16; PosnAct function_input uint16; ForkAct function_output; Fork3DirReq output uint8; Fork3SyncPha output uint8; Fork3DeltaSpdReq output uint16; Fork3PosnReq output uint16; Fork3DeltaSpdAct output uint16; Fork3Req input uint8; Fork3Act output uint8; Fork3PosnVal input uint16; Fork3ADeltaSpdAct input uint16; Fork3A parameter uint8; Fork3B parameter uint8; Fork3PosnSyncA parameter uint16; Fork3PosnSyncB parameter uint16; Fork3SyncTar parameter uint16; Fork3ReqLoc local uint8; Fork3DeltaSpdTar parameter uint16; FcnCallTime parameter uint8; Fork3PosnA parameter uint16; Fork3PosnB parameter uint16; Fork3PosnNeut parameter uint16; Fork3PosnNeutB parameter uint16; Fork3PosnNeutA parameter uint16; Fork3BDeltaSpdAct input uint16; Fork3ActLoc local uint8

== stateflow chart MIL_ASW/Application_Software_SHAW/ASW_GearPositioner/Fork4 ==
  state PosnTar = PosnTar(ForkAct) [function]
  state ForkAct = Ini_ForkAct(PosnAct) [function]
  state Initialization
    en:
    Fork4DirReq=0;
    Fork4PosnReq=Fork4PosnVal;
    du:
    Fork4ActLoc=Ini_ForkAct(Fork4PosnVal);
    ex:
    Fork4PosnReq=Fork4PosnVal;
  state error1
  state error
  state PositionBEngage
    state Phase1
      en,du:
      Fork4SyncPha=1;
      Fork4PosnReq=Fork4PosnVal-PosnTar(Fork4PosnVal);
    state Phase2
      en,du:
      Fork4SyncPha=2;
      Fork4DeltaSpdAct=Fork4BDeltaSpdAct;
      Fork4DeltaSpdReq=Fork4DeltaSpdAct-Fork4DeltaSpdTar*FcnCallTime;
    state Phase3
      en,du:
      Fork4SyncPha=3;
      Fork4PosnReq=Fork4PosnVal-PosnTar(Fork4PosnVal);
    PositionBEngage.Phase1 -> PositionBEngage.Phase2 : [Fork4PosnReq<=Fork4PosnSyncB]
    PositionBEngage.Phase2 -> PositionBEngage.Phase3 : [Fork4DeltaSpdAct<=Fork4SyncTar]
  state PositionAEngage
    state Phase1
      en,du:
      Fork4SyncPha=1;
      Fork4PosnReq=Fork4PosnVal+PosnTar(Fork4PosnVal);
    state Phase2
      en,du:
      Fork4SyncPha=2;
      Fork4DeltaSpdAct=Fork4ADeltaSpdAct;
      Fork4DeltaSpdReq=Fork4DeltaSpdAct-Fork4DeltaSpdTar*FcnCallTime;
    state Phase3
      en,du:
      Fork4SyncPha=3;
      Fork4PosnReq=Fork4PosnVal+PosnTar(Fork4PosnVal);
    PositionAEngage.Phase1 -> PositionAEngage.Phase2 : [Fork4PosnVal>=Fork4PosnSyncA]
    PositionAEngage.Phase2 -> PositionAEngage.Phase3 : [Fork4DeltaSpdAct<=Fork4SyncTar]
  state PositionADisengage
    state Phase1
      en:
      Fork4SyncPha=4;
      Fork4PosnReq=Fork4PosnNeut;
  state PositionBDisengage
    state Phase1
      en:
      Fork4SyncPha=4;
      Fork4PosnReq=Fork4PosnNeut;
  state Finish
    en:
    Fork4DirReq=0;
    Fork4ActLoc=Fork4ReqLoc;
    Fork4Act=Fork4ReqLoc;
  state Finish1
    en:
    Fork4DirReq=0;
    Fork4ActLoc=Fork4ReqLoc;
    Fork4Act=Fork4ReqLoc;
  (default) -> Initialization
  (junction 105) -> Initialization
  (junction 145) -> Initialization
  (junction 183) -> (junction 105)
  (junction 177) -> (junction 145)
  Initialization -> (junction 19) : [Fork4Req!=Fork4ActLoc]{Fork4ReqLoc=Fork4Req;}
  error -> (junction 177)
  (junction 21) -> error1 [order 3] : [Fork4ActLoc!=0]
  (junction 19) -> (junction 21) [order 2]
  (junction 19) -> (junction 22) [order 1] : [Fork4ReqLoc==0]
  (junction 22) -> error [order 3]
  error1 -> (junction 183)
  (junction 146) -> (junction 177)
  (junction 22) -> (junction 132) [order 1] : [Fork4ActLoc==Fork4A||...
      | Fork4ActLoc==Fork4A*10]
  (junction 21) -> (junction 27) [order 2] : [Fork4ReqLoc==Fork4B]
  (junction 21) -> (junction 72) [order 1] : [Fork4ReqLoc==Fork4A]
  (junction 22) -> (junction 131) [order 2] : [Fork4ActLoc==Fork4B||...
      | Fork4ActLoc==Fork4B*10]
  (junction 106) -> (junction 183)
  (junction 27) -> PositionBEngage.Phase1 : {Fork4DirReq=3;}
  (junction 131) -> PositionBDisengage.Phase1 : {Fork4DirReq=2;}
  (junction 72) -> PositionAEngage.Phase1 : {Fork4DirReq=1;}
  (junction 132) -> PositionADisengage.Phase1 : {Fork4DirReq=4;}
  Finish -> (junction 106)
  Finish1 -> (junction 146)
  PositionBEngage.Phase3 -> Finish : [Fork4PosnVal<=Fork4PosnB]
      | {Fork4SyncPha=4;}
  PositionADisengage.Phase1 -> Finish1 : [Fork4PosnVal<=Fork4PosnNeutA]
      | {Fork4SyncPha=0;}
  PositionAEngage.Phase3 -> Finish : [Fork4PosnVal>=Fork4PosnA]
      | {Fork4SyncPha=4;}
  PositionBDisengage.Phase1 -> Finish1 : [Fork4PosnVal>=Fork4PosnNeutB]
      | {Fork4SyncPha=0;}
  data: PosnTar function_output; ForkAct function_input uint16; PosnAct function_input uint16; ForkAct function_output; Fork4DirReq output uint8; Fork4SyncPha output uint8; Fork4DeltaSpdReq output uint16; Fork4PosnReq output uint16; Fork4DeltaSpdAct output uint16; Fork4Req input uint8; Fork4Act output uint8; Fork4PosnVal input uint16; Fork4ADeltaSpdAct input uint16; Fork4A parameter uint8; Fork4B parameter uint8; Fork4PosnSyncA parameter uint16; Fork4PosnSyncB parameter uint16; Fork4SyncTar parameter uint16; Fork4ReqLoc local uint8; Fork4DeltaSpdTar parameter uint16; FcnCallTime parameter uint8; Fork4PosnA parameter uint16; Fork4PosnB parameter uint16; Fork4PosnNeut parameter uint16; Fork4PosnNeutB parameter uint16; Fork4PosnNeutA parameter uint16; Fork4BDeltaSpdAct input uint16; Fork4ActLoc local uint8
